simulink model "Jacob_Edit"  (R2024b)
settings: Solver=VariableStepAuto  StartTime=0.0  StopTime=1000  RelTol=1e-3
values from neighbouring files (symbols this model uses):
  K_d = 0    [Project2_Part2_code.m]
  K_i = 0.12    [Project2_Part2_code.m]
  K_p = 2.5    [Project2_Part2_code.m]
undefined symbols (not defined in the file or in its folder): carData
settings Model: NumberOfSteps=10  Creator=dxego  LastModifiedBy=jacobcody
settings RTWCC: GPUComputeCapability=3.5

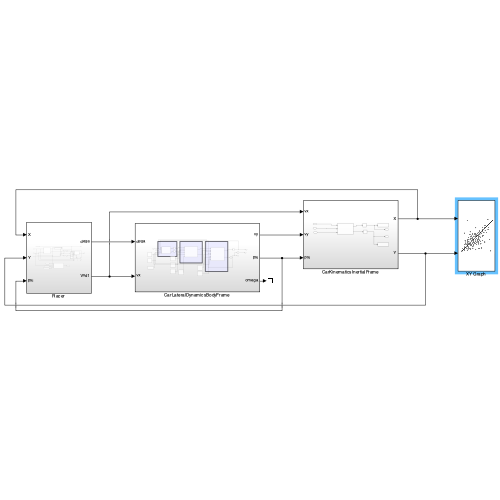
[thumbnail: Simulink's stored preview of the top-level diagram]
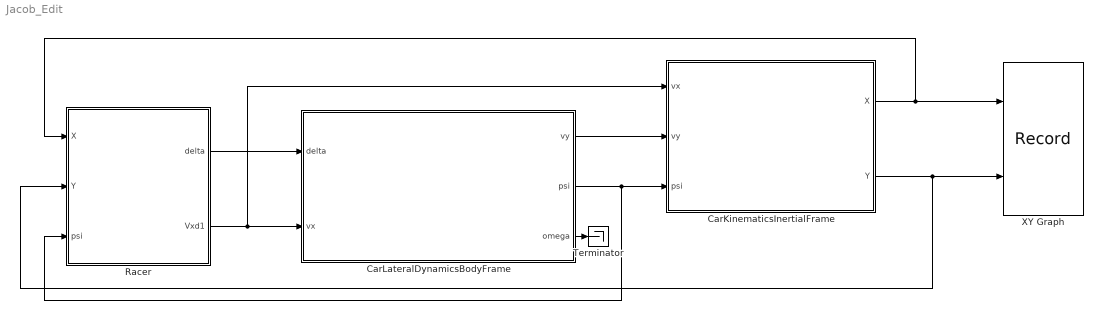
== system Jacob_Edit ==
  CarKinematicsInertialFrame : Subsystem
  CarLateralDynamicsBodyFrame : Subsystem
  Racer : Subsystem
  Terminator : Terminator
  XY Graph : Record  FileSettingsInternal="{\"entries\":[{\"content\":{\"excelSettings\":{\"content\":{},\"type\":\"Streamout.ExcelSettings\"}},\"type\":\"Streamout.FileSettingStorage\",\"uuid\":\"\"}],\"packageUris\":[\"http:\\/\\/schema.mathworks.com\\/mf0\\/streamout_blocks\\/R2020a\"],\"version\":\"1.0\"}"  Layout=[1 1]  SignalsInternal="{\"entries\":[{\"content\":{\"signals\":[{\"content\":{\"blockPath\":[],\"dimensions\":[1],\"domain\":\"\",\"lineColor\":\"#d95319\",\"plots\":[ 1 ],\"port\":1,\"sid\":[\"\"],\"signalID\":1,\"signalName\":\"CarKinematicsInertialFrame:1\"},\"type\":\"RecordBlkView.Signal\",\"uuid\":\"\"},{\"content\":{\"blockPath\":[],\"dimensions\":[1],\"domain\":\"\",\"lineColor\":\"#edb120\",\"plots\":[ 1 ],\"port\":2,\"sid\":[\"\"],\"signalID\":2,\"signalName\":\"CarKinematicsInertialFrame:2\"},\"type\":\"RecordBlkView.Signal\",\"uuid\":\"\"},{\"content\":{\"blockPath\":[],\"dimensions\":[1],\"domain\":\"\",\"lineColor\":\"#fe330a\",\"lineWidth\":2,\"port\":1,\"sid\":[\"\"],\"signalID\":3,\"signalName\":\"Integrator\"},\"type\":\"RecordBlkView.Signal\",\"uuid\":\"\"},{\"content\":{\"blockPath\":[],\"dimensions\":[1],\"domain\":\"\",\"lineColor\":\"#22b573\",\"lineWidth\":2,\"port\":1,\"sid\":[\"\"],\"signalID\":4,\"signalName\":\"Integrator1\"},\"type\":\"RecordBlkView.Signal\",\"uuid\":\"\"},{\"content\":{\"blockPath\":[],\"dimensions\":[1],\"domain\":\"\",\"lineColor\":\"#0072bd\",\"lineWidth\":2,\"port\":1,\"sid\":[\"\"],\"signalID\":5,\"signalName\":\"Lateral Control Function\"},\"type\":\"RecordBlkView.Signal\",\"uuid\":\"\"}]},\"type\":\"RecordBlkView.InputSignals\",\"uuid\":\"\"}],\"packageUris\":[\"http:\\/\\/schema.mathworks.com\\/mf0\\/streamout_blocks\\/R2020a\"],\"version\":\"1.0\"}"  VisualizationBindings="{\"xyplotplugin\":{\"info\":[{\"series\":[{\"bindingParametersList\":[{\"parameter\":\"X-Axis\",\"signalID\":1,\"signalName\":\"CarKinematicsInertialFrame:1\"},{\"parameter\":\"Y-Axis\",\"signalID\":2,\"signalName\":\"CarKinematicsInertialFrame:2\"}],\"seriesID\":0}],\"subplotID\":1}]}}"  CompatibilityTag=XY  st=-1
  wires:
  Racer/1(delta) -> CarLateralDynamicsBodyFrame/1(delta)
  CarLateralDynamicsBodyFrame/1(vy) -> CarKinematicsInertialFrame/2(vy)
  CarLateralDynamicsBodyFrame/2(psi) -> Racer/3(psi), CarKinematicsInertialFrame/3(psi)
  CarKinematicsInertialFrame/1(X) -> Racer/1(X), XY Graph/1
  CarKinematicsInertialFrame/2(Y) -> Racer/2(Y), XY Graph/2
  Racer/2(Vxd1) -> CarKinematicsInertialFrame/1(vx), CarLateralDynamicsBodyFrame/2(vx)
  CarLateralDynamicsBodyFrame/3(omega) -> Terminator/1

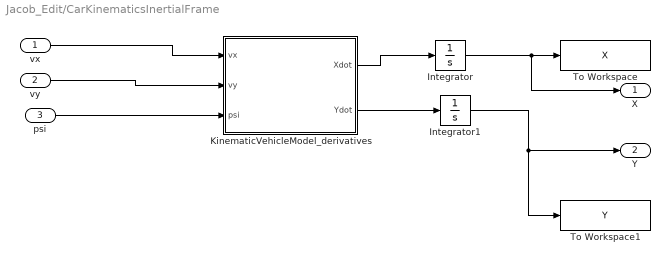
== system Jacob_Edit/CarKinematicsInertialFrame ==
  vx : Inport
  vy : Inport  Port=2
  psi : Inport  Port=3
  Integrator : Integrator  InitialCondition=carData.init.X0
  Integrator1 : Integrator  InitialCondition=carData.init.Y0
  KinematicVehicleModel_derivatives : MATLAB Function  TreatAsAtomicUnit=on
  To Workspace : ToWorkspace  VariableName=X  SaveFormat=Timeseries  SampleTime=-1
  To Workspace1 : ToWorkspace  VariableName=Y  SaveFormat=Timeseries  SampleTime=-1
  X : Outport
  Y : Outport  Port=2
  wires:
  Integrator/1 -> X/1, To Workspace/1
  Integrator1/1 -> To Workspace1/1, Y/1
  vx/1 -> KinematicVehicleModel_derivatives/1(vx)
  vy/1 -> KinematicVehicleModel_derivatives/2(vy)
  psi/1 -> KinematicVehicleModel_derivatives/3(psi)
  KinematicVehicleModel_derivatives/1(Xdot) -> Integrator/1
  KinematicVehicleModel_derivatives/2(Ydot) -> Integrator1/1

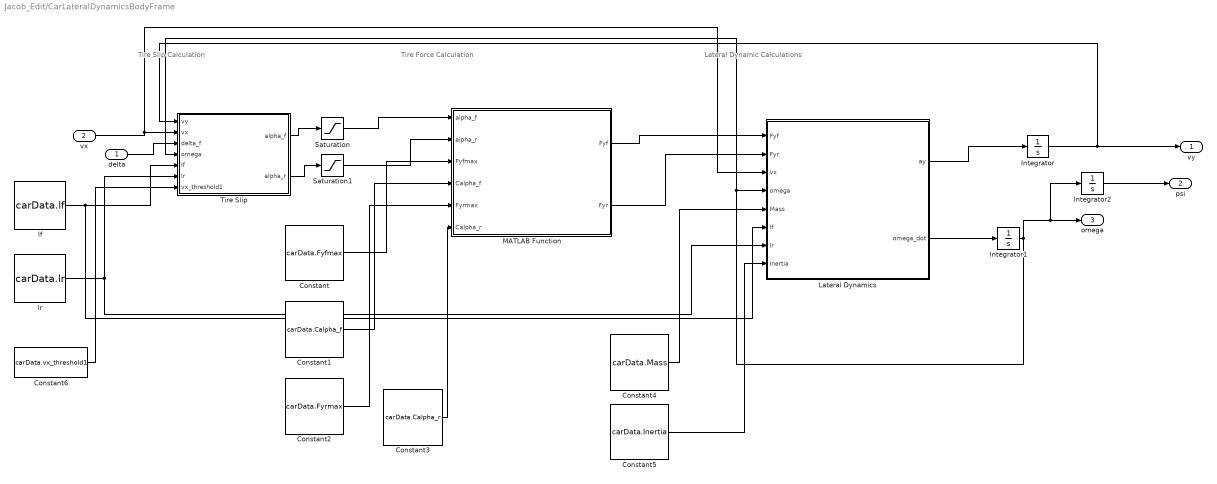
== system Jacob_Edit/CarLateralDynamicsBodyFrame ==
  note: Tire Slip Calculation
  note: Tire Force Calculation
  note: Lateral Dynamic Calculations
  delta : Inport
  vx : Inport  Port=2
  Constant : Constant  Value=carData.Fyfmax
  Constant1 : Constant  Value=carData.Calpha_f
  Constant2 : Constant  Value=carData.Fyrmax
  Constant3 : Constant  Value=carData.Calpha_r
  Constant4 : Constant  Value=carData.Mass
  Constant5 : Constant  Value=carData.Inertia
  Constant6 : Constant  Value=carData.vx_threshold1
  Integrator : Integrator  InitialCondition=carData.init.vy0
  Integrator1 : Integrator  InitialCondition=carData.init.omega0
  Integrator2 : Integrator  InitialCondition=carData.init.psi0  WrappedStateUpperValue=2*pi  WrappedStateLowerValue=0
  Lateral Dynamics : MATLAB Function  TreatAsAtomicUnit=on
  MATLAB Function : MATLAB Function  TreatAsAtomicUnit=on
  Saturation : Saturate  UpperLimit=carData.maxAlpha  LowerLimit=-carData.maxAlpha
  Saturation1 : Saturate  UpperLimit=carData.maxAlpha  LowerLimit=-carData.maxAlpha
  "Tire Slip " : MATLAB Function  TreatAsAtomicUnit=on
  lf : Constant  Value=carData.lf
  lr : Constant  Value=carData.lr
  vy : Outport
  psi : Outport  Port=2
  omega : Outport  Port=3
  wires:
  Lateral Dynamics/1(ay) -> Integrator/1
  Integrator/1 -> "Tire Slip "/1(vy), vy/1
  Lateral Dynamics/2(omega_dot) -> Integrator1/1
  Integrator1/1 -> Integrator2/1, omega/1, Lateral Dynamics/4(omega), "Tire Slip "/4(omega)
  "Tire Slip "/1(alpha_f) -> Saturation/1
  Saturation/1 -> MATLAB Function/1(alpha_f)
  Saturation1/1 -> MATLAB Function/2(alpha_r)
  vx/1 -> Lateral Dynamics/3(vx), "Tire Slip "/2(vx)
  delta/1 -> "Tire Slip "/3(delta_f)
  Integrator2/1 -> psi/1
  "Tire Slip "/2(alpha_r) -> Saturation1/1
  MATLAB Function/1(Fyf) -> Lateral Dynamics/1(Fyf)
  MATLAB Function/2(Fyr) -> Lateral Dynamics/2(Fyr)
  lf/1 -> Lateral Dynamics/6(lf), "Tire Slip "/5(lf)
  lr/1 -> Lateral Dynamics/7(lr), "Tire Slip "/6(lr)
  Constant/1 -> MATLAB Function/3(Fyfmax)
  Constant1/1 -> MATLAB Function/4(Calpha_f)
  Constant2/1 -> MATLAB Function/5(Fyrmax)
  Constant3/1 -> MATLAB Function/6(Calpha_r)
  Constant4/1 -> Lateral Dynamics/5(Mass)
  Constant5/1 -> Lateral Dynamics/8(Inertia)
  Constant6/1 -> "Tire Slip "/7(vx_threshold1)

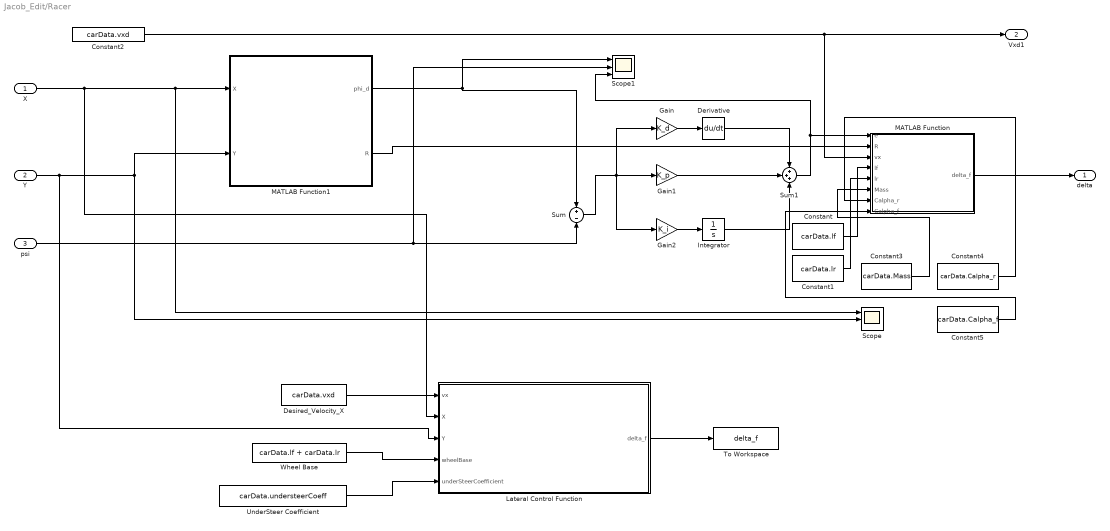
== system Jacob_Edit/Racer ==
  X : Inport
  Y : Inport  Port=2
  psi : Inport  Port=3
  Constant : Constant  Value=carData.lf
  Constant1 : Constant  Value=carData.lr
  Constant2 : Constant  Value=carData.vxd
  Constant3 : Constant  Value=carData.Mass
  Constant4 : Constant  Value=carData.Calpha_r
  Constant5 : Constant  Value=carData.Calpha_f
  Derivative : Derivative
  Desired_Velocity_X : Constant  Value=carData.vxd
  Gain : Gain  Gain=K_d
  Gain1 : Gain  Gain=K_p
  Gain2 : Gain  Gain=K_i
  Integrator : Integrator
  Lateral Control Function : MATLAB Function  TreatAsAtomicUnit=on
  MATLAB Function : MATLAB Function  TreatAsAtomicUnit=on
  MATLAB Function1 : MATLAB Function  TreatAsAtomicUnit=on
  Scope : Scope  NumInputPorts=3
  Scope1 : Scope  NumInputPorts=3
  Sum : Sum  Inputs=+-
  Sum1 : Sum  Inputs=+++
  To Workspace : ToWorkspace  VariableName=delta_f  SaveFormat=Timeseries  SampleTime=-1
  UnderSteer Coefficient : Constant  Value=carData.understeerCoeff
  Wheel Base : Constant  Value=carData.lf + carData.lr
  delta : Outport
  Vxd1 : Outport  Port=2
  wires:
  Constant2/1 -> MATLAB Function/3(vx), Vxd1/1
  Y/1 -> Lateral Control Function/3(Y), MATLAB Function1/2(Y), Scope/2
  psi/1 -> Scope1/2, Sum/2
  MATLAB Function/1(delta_f) -> delta/1
  Gain/1 -> Derivative/1
  Gain2/1 -> Integrator/1
  Sum/1 -> Gain2/1, Gain/1, Gain1/1
  Derivative/1 -> Sum1/1
  Gain1/1 -> Sum1/2
  Integrator/1 -> Sum1/3
  Sum1/1 -> MATLAB Function/1(e), Scope1/3
  MATLAB Function1/1(phi_d) -> Sum/1, Scope1/1
  MATLAB Function1/2(R) -> MATLAB Function/2(R)
  X/1 -> Lateral Control Function/2(X), MATLAB Function1/1(X), Scope/1
  Lateral Control Function/1(delta_f) -> To Workspace/1
  Desired_Velocity_X/1 -> Lateral Control Function/1(vx)
  Wheel Base/1 -> Lateral Control Function/4(wheelBase)
  UnderSteer Coefficient/1 -> Lateral Control Function/5(underSteerCoefficient)
  Constant/1 -> MATLAB Function/4(lf)
  Constant1/1 -> MATLAB Function/5(lr)
  Constant3/1 -> MATLAB Function/6(Mass)
  Constant4/1 -> MATLAB Function/7(Calpha_r)
  Constant5/1 -> MATLAB Function/8(Calpha_f)

== matlab function Jacob_Edit/CarLateralDynamicsBodyFrame/Tire Slip  ==
  data: vy input; alpha_f output; vx input; delta_f input; omega input; lf input; alpha_r output; lr input; vx_threshold1 input
function [alpha_f, alpha_r] = fcn(vy,  vx, delta_f, omega, lf, lr, vx_threshold1)


if abs(vx)> vx_threshold1
      alpha_f = delta_f - (vy + omega * lf) / vx;
      alpha_r = - (vy - omega * lr) / vx;
else
      alpha_f = 0;
      alpha_r = 0;
end



end

== matlab function Jacob_Edit/Racer/MATLAB Function1 ==
  data: X input; phi_d output; Y input; R output
function [phi_d , R] = desired_head(X,Y)
phi_d = 0;
R = 0;
%===============================
if X>900 && Y<200
    phi_d = (2*pi()) - acos((X-900)/200) -deg2rad(270);
    R = 200;
elseif X>900 && Y>=200
    phi_d = acos((X-900)/200) + deg2rad(90);
    R = 200;
elseif 0 <= X && X <= 900 && Y >200
    phi_d = pi();
    R = 0;
elseif X < 0 && Y >= 200
    phi_d = (2*pi()) - acos(-X/200) - deg2rad(90);
    R = 200;
elseif X < 0 && Y <200
    phi_d = acos(-X/200) + deg2rad(270);
    R = 200;
elseif X <= 900 && Y < 200 && X >= 0
    phi_d = 0;
    R = 0;
end

phi_d = unwrap(phi_d);

phi_d = mod(phi_d, 2*pi());

%===============================
% if X > 900
%     delta = 5;
% elseif X < 0
%     delta = -5;
% else
%     delta = 0;
% end

%===============================
% if X > 900
%     delta = 5;
% elseif X < 0
%     delta = 5;
% else
%     delta = 0;
% end

== matlab function Jacob_Edit/Racer/Lateral Control Function ==
  data: vx input; delta_f output; X input; Y input; wheelBase input; underSteerCoefficient input
function delta_f   = latControl(vx,X,Y,wheelBase, underSteerCoefficient)

track_radius = 200;
track_length = 900;

track_seg1_x0 = 0;
track_seg1_y0 = 0;
track_seg1_x1 = track_length;
track_seg1_y1 = 0;
track_seg2_x0 = track_seg1_x1;
track_seg2_y0 = track_seg1_y1;
track_seg2_x1 = track_seg2_x0;
track_seg2_y1 = track_seg2_y0 + 2 * track_radius;
track_seg3_x0 = track_seg2_x1;
track_seg3_y0 = track_seg2_y1;
track_seg3_x1 = track_seg3_x0 - track_length;
track_seg3_y1 = track_seg3_y0;
track_seg4_x0 = track_seg3_x1;
track_seg4_y0 = track_seg3_y1;
track_seg4_x1 = track_seg1_x0;
track_seg4_y1 = track_seg1_y0;

if X > track_seg1_x0
    if X > track_seg1_x1
        segment = 2;
    else
        if Y > (track_seg2_y0 + track_seg2_y1)/2
            segment = 3;
        else
            segment = 1;
        end
    end
else
    segment = 4;
end



switch(segment)
    case 1
        delta_f = 0;
    case 2
        delta_f = - (wheelBase / track_radius + 1 * underSteerCoefficient * vx^2);
    case 3
        delta_f = 0;
    case 4
        delta_f = - (wheelBase / track_radius + 1 * underSteerCoefficient * vx^2);
    otherwise
        delta_f = 0;
end
function y = fcn(u)

y = u;

== matlab function Jacob_Edit/CarKinematicsInertialFrame/KinematicVehicleModel_derivatives ==
  data: vx input; Xdot output; vy input; psi input; Ydot output
function [Xdot, Ydot] = fcn(vx, vy, psi)
    temp = TF(psi) * [vx;vy]; 
    Xdot = temp(1);
    Ydot = temp(2);
  
end

function y = TF(psi)
    y = [cos(psi), -sin(psi); sin(psi), cos(psi)];
end

== matlab function Jacob_Edit/CarLateralDynamicsBodyFrame/MATLAB Function ==
  data: alpha_f input; Fyf output; alpha_r input; Fyfmax input; Fyr output; Calpha_f input; Fyrmax input; Calpha_r input
function [Fyf, Fyr] = fcn(alpha_f, alpha_r, Fyfmax, Calpha_f, Fyrmax, Calpha_r)

Fyf = min(Fyfmax,Calpha_f * alpha_f);
Fyr = min(Fyrmax, Calpha_r * alpha_r);

end

== matlab function Jacob_Edit/CarLateralDynamicsBodyFrame/Lateral Dynamics ==
  data: Fyf input; ay output; Fyr input; vx input; omega input; Mass input; omega_dot output; lf input; lr input; Inertia input
function [ay, omega_dot] = fcn(Fyf, Fyr, vx, omega, Mass, lf, lr, Inertia)

Fy = Fyf + Fyr;
ay = Fy / Mass - omega * vx;
        
M  = Fyf * lf - Fyr *lr;        
omega_dot = M / Inertia;        

end

== matlab function Jacob_Edit/Racer/MATLAB Function ==
  data: e input; delta_f output; R input; vx input; lf input; lr input; Mass input; Calpha_r input; Calpha_f input
function delta_f = fcn(e, R, vx, lf, lr, Mass, Calpha_r, Calpha_f)
L = lr + lf;
if R ~= 0
    delta_f = e + (L/R)+((Mass/(L*R))*((lr/Calpha_r)-(lf/Calpha_f))*(vx^2));
else
    delta_f = e;

end
